simulink model "de_dsb"  (R2016a)
settings: Solver=VariableStepAuto  StartTime=0.0  StopTime=20.0  RelTol=1e-3
libraries: simulink x2, dsparch4 x1
settings Model: Creator=iP Store  LastModifiedBy=iP Store

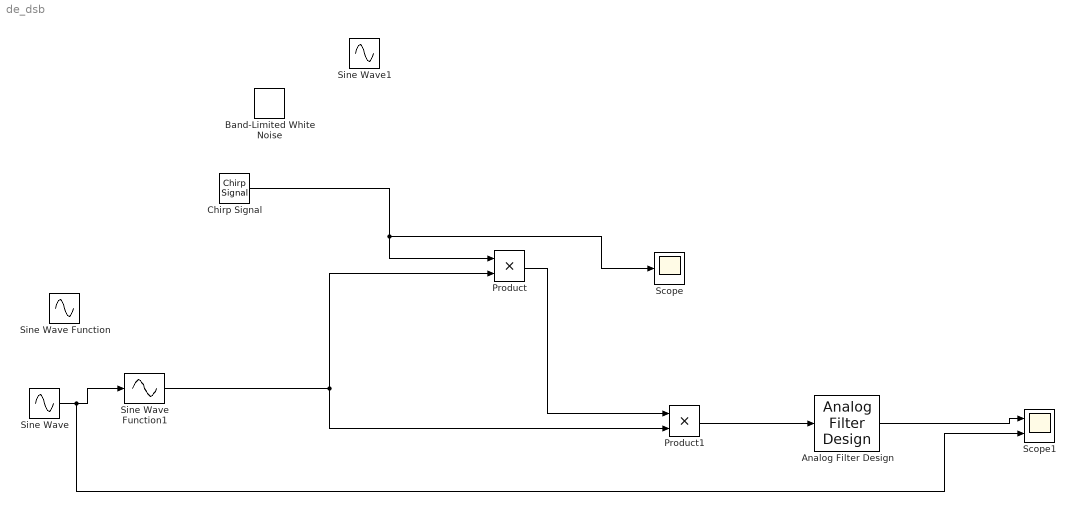
== system de_dsb ==
  Analog Filter Design : dsparch4/Analog Filter Design  method=Butterworth  filttype=Lowpass  N=10  Wlo=200  Whi=80  Rp=2  Rs=40
  Band-Limited White Noise : simulink/Sources/Band-Limited White Noise  Cov=[0.1]  Ts=0.1  seed=[23341]
  Chirp Signal : simulink/Sources/Chirp Signal  f1=0.1  T=100  f2=4
  Product : Product
  Product1 : Product
  Scope : Scope
  Scope1 : Scope  NumInputPorts=2
  Sine Wave : Sin  Frequency=2*pi  SampleTime=0
  Sine Wave Function : Sin  TimeSource=Use external signal  Amplitude=5  Phase=pi/2  SampleTime=0
  Sine Wave Function1 : Sin  TimeSource=Use external signal  Frequency=1e+3  SampleTime=0
  Sine Wave1 : Sin  Amplitude=4  Frequency=100  SampleTime=0
  wires:
  Sine Wave/1 -> Scope1/2, Sine Wave Function1/1
  Sine Wave Function1/1 -> Product/2, Product1/2
  Product/1 -> Product1/1
  Product1/1 -> Analog Filter Design/1
  Analog Filter Design/1 -> Scope1/1
  Chirp Signal/1 -> Scope/1, Product/1
